simulink model "PMLM_RESO_2017a"  (R2017a)
settings: Solver=ode14x  StartTime=0.0  StopTime=10.0  FixedStep=0.001  RelTol=1e-3
values from neighbouring files (symbols this model uses):
  a1 = (D + Kf*Ke/R)/M    (= 178.108465608)    [Para.m]
  b0 = Kf/(M*R)    (= 1.43298059965)    [Para.m]
  beta1 = 2*wo    (= 2000)    [Para.m]
  beta2 = wo^2    (= 1000000)    [Para.m]
  Flm = 100    [Para.m]
  kd = 2*wc    (= 1000)    [Para.m]
  kp = wc^2    (= 250000)    [Para.m]
  M = 5.4    [Para.m]
  wt = 50    [Para.m]
settings Model: Creator=chengqian  LastModifiedBy=chengqian
settings SFSimCC: SimUseLocalCustomCode=on
settings RTWCC: RTWUseLocalCustomCode=on

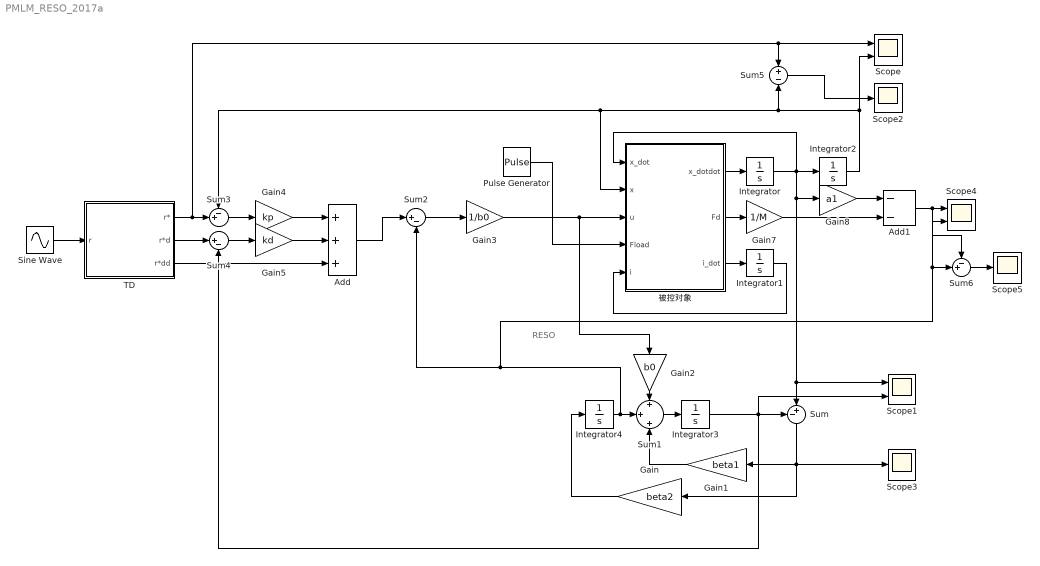
== system PMLM_RESO_2017a ==
  note: RESO
  Add : Sum  Inputs=+++
  Add1 : Sum  Inputs=--
  Gain : Gain  Gain=beta2
  Gain1 : Gain  Gain=beta1
  Gain2 : Gain  Gain=b0
  Gain3 : Gain  Gain=1/b0
  Gain4 : Gain  Gain=kp
  Gain5 : Gain  Gain=kd
  Gain7 : Gain  Gain=1/M
  Gain8 : Gain  Gain=a1
  Integrator{,1..4} (5 alike) : Integrator
  Pulse Generator : DiscretePulseGenerator  PulseType=Time based  Amplitude=Flm*10  Period=3  PulseWidth=20
  Scope : Scope  NumInputPorts=2
  Scope1 : Scope  NumInputPorts=2
  Scope2 : Scope
  Scope3 : Scope
  Scope4 : Scope  NumInputPorts=2
  Scope5 : Scope
  Sine Wave : Sin  Amplitude=100  SampleTime=0
  Sum : Sum  Inputs=-+|
  Sum1 : Sum  Inputs=+|+|+
  Sum2 : Sum  Inputs=|+-
  Sum3 : Sum  Inputs=-+|
  Sum4 : Sum  Inputs=|+-
  Sum5 : Sum  Inputs=+|-
  Sum6 : Sum  Inputs=-+|
  TD : Subsystem
  被控对象 : MATLAB Function  TreatAsAtomicUnit=on
  wires:
  被控对象/1(x_dotdot) -> Integrator/1
  被控对象/3(i_dot) -> Integrator1/1
  Integrator1/1 -> 被控对象/5(i)
  Integrator/1 -> 被控对象/1(x_dot), Integrator2/1, Gain8/1, Scope1/1, Sum/2
  Integrator3/1 -> Sum/1, Scope1/2, Sum4/2
  Gain/1 -> Integrator4/1
  Sum1/1 -> Integrator3/1
  Integrator4/1 -> Sum1/2, Scope4/2, Sum6/2, Sum2/2
  Gain1/1 -> Sum1/3
  Gain2/1 -> Sum1/1
  Sum2/1 -> Gain3/1
  Gain3/1 -> Gain2/1, 被控对象/3(u)
  Sine Wave/1 -> TD/1(r)
  TD/1(r*) -> Sum5/1, Scope/1, Sum3/2
  Sum3/1 -> Gain4/1
  TD/2(r*d) -> Sum4/1
  Sum4/1 -> Gain5/1
  Gain4/1 -> Add/1
  Gain5/1 -> Add/2
  TD/3(r*dd) -> Add/3
  Add/1 -> Sum2/1
  Pulse Generator/1 -> 被控对象/4(Fload)
  Integrator2/1 -> Scope/2, Sum5/2, Sum3/1, 被控对象/2(x)
  Sum5/1 -> Scope2/1
  Sum/1 -> Scope3/1, Gain1/1, Gain/1
  被控对象/2(Fd) -> Gain7/1
  Gain7/1 -> Add1/2
  Gain8/1 -> Add1/1
  Add1/1 -> Scope4/1, Sum6/1
  Sum6/1 -> Scope5/1

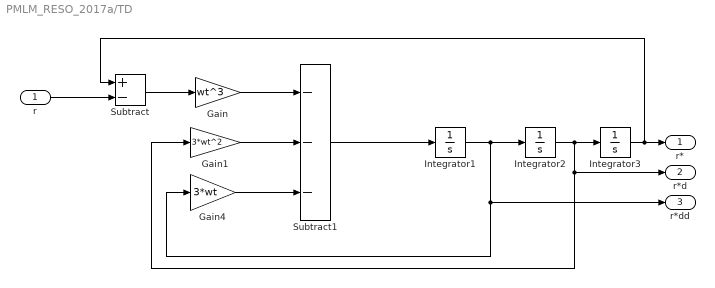
== system PMLM_RESO_2017a/TD ==
  r : Inport
  Gain : Gain  Gain=wt^3
  Gain1 : Gain  Gain=3*wt^2
  Gain4 : Gain  Gain=3*wt
  Integrator1 : Integrator
  Integrator2 : Integrator
  Integrator3 : Integrator
  Subtract : Sum  Inputs=+-
  Subtract1 : Sum  Inputs=---
  r* : Outport
  r*d : Outport  Port=2
  r*dd : Outport  Port=3
  wires:
  Integrator2/1 -> Integrator3/1, Gain1/1, r*d/1
  Gain1/1 -> Subtract1/2
  Subtract/1 -> Gain/1
  Gain/1 -> Subtract1/1
  Integrator3/1 -> Subtract/1, r*/1
  Gain4/1 -> Subtract1/3
  Subtract1/1 -> Integrator1/1
  Integrator1/1 -> Gain4/1, r*dd/1, Integrator2/1
  r/1 -> Subtract/2

== matlab function PMLM_RESO_2017a/被控对象 ==
  data: x_dot input; x_dotdot output; Fd output; x input; u input; Fload input; i input; i_dot output
function [x_dotdot,Fd,i_dot] = fcn(x_dot,x,u,Fload,i)

%%PMLM 参数
M = 5.4;
D = 10;
R = 16.8;
L = 17.4*0.001;
Kf = 130;
Ke = 123;
Fc = 10;
Fs = 20;
Fv = 10;
Ar = 8.5;
a = 314;
phi = 0.05*pi;
Flm = 100;
xs = 0.1;

%% 控制系数 b0 = Kf/(M*R);

%%总扰动构成
Fripple = Ar*sin(a*x + phi);
Ffric = (Fc+(Fs - Fc)*exp(-(x_dot/xs)^2) + Fv*abs(x_dot))*sign(x_dot);
Fd = Fload + Fripple + Ffric;
%%模型微分方程
i_dot = (u - R*i - Ke*x_dot)/L;
x_dotdot = (Kf*i - D*x_dot - Fd)/M;
